simulink model "output_mdl"  (R2021b)
settings: Solver=ode1  StartTime=0.0  StopTime=5  FixedStep=0.0001  MaxStep=0.01  MinStep=0.001  RelTol=1e-3
values from neighbouring files (symbols this model uses):
  A = [0 1; 0 0]    [pendulum_data.m]
  B = [0;1]    [pendulum_data.m]
  C = C([1,3],:)    [comp_data.m]    (also in pendulum_data.m = [1 1])
  gamma0 = -0.5    [output_data.m]
  rho = 1    [comp_data.m]    (also in obsint_data.m; obsmod_data.m; outmod_data.m; outmodc_data.m)
  x0 = zeros(1,n)    [comp_data.m]    (also in obsint_data.m; obsmod_data.m; outmod_data.m; outmodc_data.m)
undefined symbols (not defined in the file or in its folder): F, m, p
settings Model: Creator=w.schwamm  LastModifiedBy=w.schwamm
settings DataIOCC: SaveState=on  SaveTime=off  ReturnWorkspaceOutputs=off  StateSaveName=x  TimeSaveName=t  OutputSaveName=y

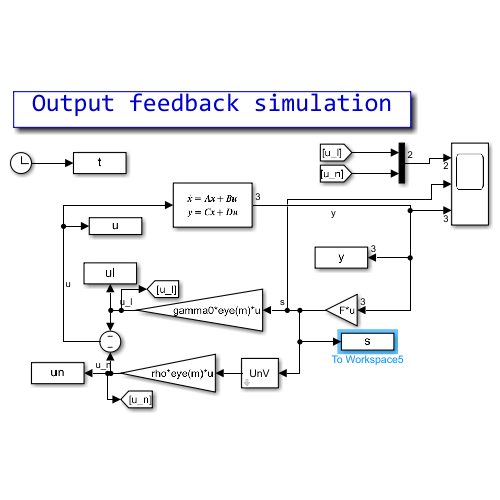
[thumbnail: Simulink's stored preview of the top-level diagram]
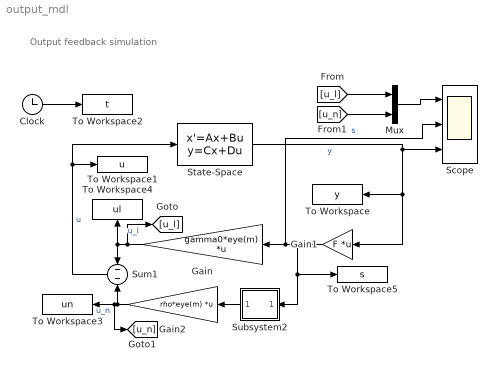
== system output_mdl ==
  note: Output feedback simulation
  Clock : Clock
  Gain : Gain  Gain=gamma0*eye(m)  Multiplication=Matrix(K*u)
  Gain1 : Gain  Gain=F  Multiplication=Matrix(K*u)
  Gain2 : Gain  Gain=rho*eye(m)  Multiplication=Matrix(K*u)
  Mux : Mux  Inputs=2
  Scope : Scope  NumInputPorts=3
  State-Space : StateSpace  A=A  B=B  C=C  D=zeros(p,m)  InitialCondition=x0
  Subsystem2 : Subsystem  mask{delta=0.001}
      mask prompts: delta "Unit vector delta:"
      mask Display: disp('UnV')
  Sum1 : Sum  Inputs=--
  To Workspace : ToWorkspace  VariableName=y  SaveFormat=Timeseries  SampleTime=-1
      settings: MaxDataPoints=1000000
  To Workspace1 : ToWorkspace  VariableName=u  SaveFormat=Timeseries  SampleTime=-1
      settings: MaxDataPoints=1000000
  To Workspace2 : ToWorkspace  VariableName=t  SaveFormat=Timeseries  SampleTime=-1
      settings: MaxDataPoints=1000000
  To Workspace3 : ToWorkspace  VariableName=un  SaveFormat=Timeseries  SampleTime=-1
      settings: MaxDataPoints=1000000
  To Workspace4 : ToWorkspace  VariableName=ul  SaveFormat=Timeseries  SampleTime=-1
      settings: MaxDataPoints=1000000
  To Workspace5 : ToWorkspace  VariableName=s  SaveFormat=Timeseries  SampleTime=-1
      settings: MaxDataPoints=1000000
  wires:
  Sum1/1 -> State-Space/1, To Workspace1/1  "u"
  Clock/1 -> To Workspace2/1
  Subsystem2/1(Out1) -> Gain2/1
  Gain2/1 -> Sum1/2, [u_n], To Workspace3/1  "u_n"
  Gain/1 -> [u_l], To Workspace4/1, Sum1/1  "u_l"
  Gain1/1 -> To Workspace5/1, Subsystem2/1(In1), Scope/2, Gain/1  "s"
  State-Space/1 -> Scope/3, Gain1/1, To Workspace/1  "y"
  Mux/1 -> Scope/1
  [u_l] -> Mux/1
  [u_n] -> Mux/2

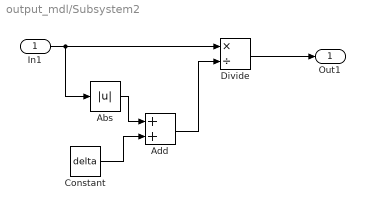
== system output_mdl/Subsystem2 ==
  In1 : Inport
  Abs : Abs
  Add : Sum
  Constant : Constant  Value=delta  SampleTime=-1
  Divide : Product  Inputs=*/
  Out1 : Outport
  wires:
  Constant/1 -> Add/2
  Add/1 -> Divide/2
  Abs/1 -> Add/1
  Divide/1 -> Out1/1
  In1/1 -> Divide/1, Abs/1
